simulink model "CIM_HA_Basic"  (R2016b)
settings: Solver=FixedStepDiscrete  StartTime=0.0  StopTime=10.0  FixedStep=TimeSteps.ModelStep  RelTol=1e-3
InitFcn:
  | BusInit;
undefined symbols (not defined in the file): Mechanical, Motor, TimeSteps
libraries: simulink x1
settings Model: Creator=KIRTACA  LastModifiedBy=KIRTACA

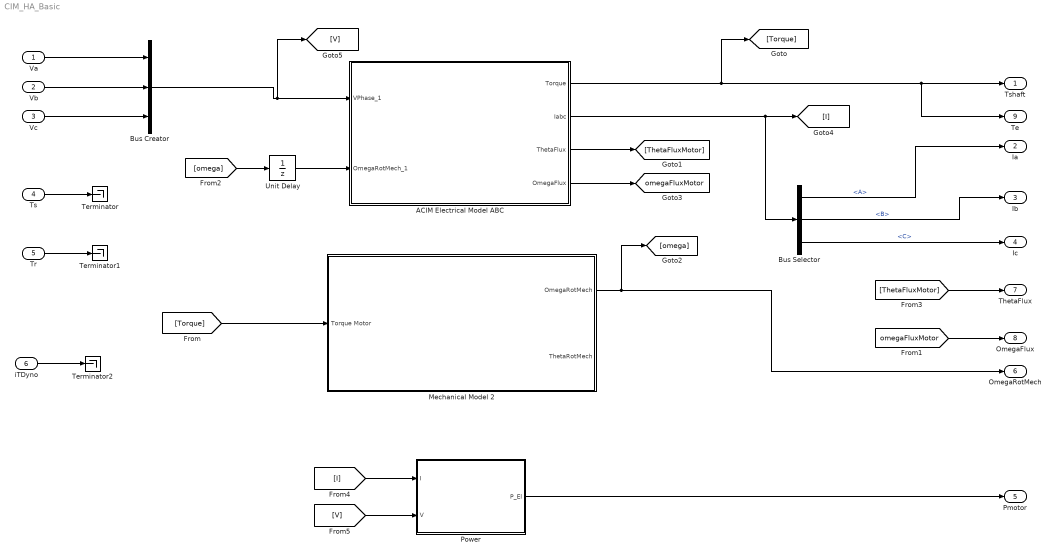
== system CIM_HA_Basic ==
  Va : Inport
  Vb : Inport  Port=2
  Vc : Inport  Port=3
  Ts : Inport  Port=4
  Tr : Inport  Port=5
  iTDyno : Inport  Port=6
  "ACIM Electrical Model ABC " : Subsystem  SystemSampleTime=Ts1  mask(ACIM_ABC){Rs=(Motor.Electrical.Rs)/(Motor.Electrical.Conn), Rr=(Motor.Electrical.Rr)/(Motor.Electrical.Conn), Ls=(Motor.Electrical.Ls)/(Motor.Electrical.Conn), Lr=(Motor.Electrical.Lr)/(Motor.Electrical.Conn), Lm=(Motor.Electrical.Lm)/(Motor.Electrical.Conn), p=Motor.Electrical.p, Ts=TimeSteps.ModelStep, Ts1=0.000125}
      mask prompts: Rs "Rs [Ohm]"; Rr "Rr [Ohm]"; Ls "Ls [H]"; Lr "Lr [H]"; Lm "Lm [H]"; Ts "Sample Time [s]"; Ts1 "Simulink:blkprm_prompts:AllBlksSampleTime"
      mask help:
      | The block implements the ACIM Electrical Model equations.
      | Input:
      | -Vphase_1: voltages applied to the motor;
      | -OmegaRotMech: mechanical rotor rotational speed;
      | Output:
      | -Torque: motor torque;
      | -Iabc: motor measured currents;
      | -OmegaFlux:
      | -ThetaFlux: angle obtained from OmegaFlux
      mask init:
      | params.Rs = Rs;
      | params.Rr = Rr;
      | params.Ls = Ls;
      | params.Lr = Lr;
      | params.Lm = Lm;
      | params.p  = p;
      | params.Ts = Ts;
      | 
      | TsACIM_ABC = Ts;
      mask Help: file:///C:\MotorControlLibrary\help/ACIM_ABC.html
      mask TypeOptions Ts1: SystemSampleTime
      mask Callback Ts1: set_param(gcb,'Ts1',num2str(eval(get_param(gcb,'Ts'))));
      mask DialogControl DescGroupVar Prompt: ACIM Electrical Model (ABC-Axis)
      mask DialogControl DescTextVar Prompt: %<MaskDescription
  Bus Creator : BusCreator  Inputs=3
  Bus Selector : BusSelector  OutputSignals=A,B,C
  Mechanical Model 2 : Subsystem  mask{TR=Motor.Mechanical.TR, M_D=Mechanical.M_D, M=Mechanical.M, R_J=Mechanical.R_J, R_Drum=Mechanical.R_Drum, InitialSpeed=0, InitialPosition=0, M_Cr=Mechanical.m_unb, R_Cr=Mechanical.r_unb, Ad=(Mechanical.damp*2*pi()*1000)/60, Ts=TimeSteps.ModelStep}
      mask prompts: TR "Transmission Ratio"; M_D "Weight Drum [Kg]"; M "Weight Inertial mass [Kg]"; R_J "Thick Inertial mass [m]"; R_Drum "Drum Radius [m]"; InitialSpeed "Initial Speed  [rad/s]"; InitialPosition "Initial Position [del_el]"; M_Cr "Weight Unbalance Load [Kg]"; R_Cr "Radius Unbalance Load [m]"; Ad "Dynamic Friction [Nm/rpm_D*1000]"; Ts "Ts [s]"
      mask init:
      | params.J = 1/2*(M_D+M)*(R_Drum^2 + (R_Drum-R_J)^2);
      | params.Ts = Ts;
      | J = 1/2*(M_D+M)*(R_Drum^2 + (R_Drum-R_J)^2);
  Power : MATLAB Function  TreatAsAtomicUnit=on
  Terminator : Terminator
  Terminator1 : Terminator
  Terminator2 : Terminator
  Unit Delay : UnitDelay  SampleTime=-1
  Tshaft : Outport
  Ia : Outport  Port=2
  Ib : Outport  Port=3
  Ic : Outport  Port=4
  Pmotor : Outport  Port=5
  OmegaRotMech : Outport  Port=6
  ThetaFlux : Outport  Port=7
  OmegaFlux : Outport  Port=8
  Te : Outport  Port=9
  tag scope: omegaFluxMotor=global
  wires:
  [Torque] -> Mechanical Model 2/1(Torque Motor)
  Mechanical Model 2/1(OmegaRotMech) -> [omega], OmegaRotMech/1
  Va/1 -> Bus Creator/1
  Vb/1 -> Bus Creator/2
  Vc/1 -> Bus Creator/3
  Ts/1 -> Terminator/1
  Tr/1 -> Terminator1/1
  Bus Selector/1 -> Ia/1  "<A>"
  Bus Selector/2 -> Ib/1  "<B>"
  Bus Selector/3 -> Ic/1  "<C>"
  [ThetaFluxMotor] -> ThetaFlux/1
  [omegaFluxMotor] -> OmegaFlux/1
  Power/1(P_El) -> Pmotor/1
  [I] -> Power/1(I)
  [V] -> Power/2(V)
  Bus Creator/1 -> [V], "ACIM Electrical Model ABC "/1(VPhase_1)
  "ACIM Electrical Model ABC "/1(Torque) -> [Torque], Te/1, Tshaft/1
  "ACIM Electrical Model ABC "/2(Iabc) -> [I], Bus Selector/1
  "ACIM Electrical Model ABC "/3(ThetaFlux) -> [ThetaFluxMotor]
  "ACIM Electrical Model ABC "/4(OmegaFlux) -> [omegaFluxMotor]
  iTDyno/1 -> Terminator2/1
  Unit Delay/1 -> "ACIM Electrical Model ABC "/2(OmegaRotMech_1)
  [omega] -> Unit Delay/1

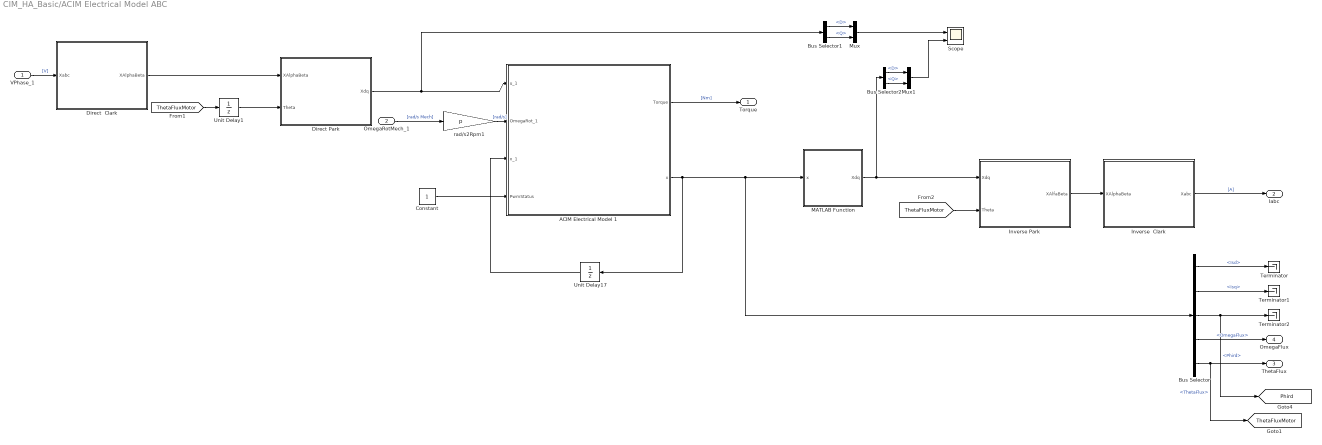
== system CIM_HA_Basic/ACIM Electrical Model ABC  ==
  VPhase_1 : Inport  OutDataTypeStr=Bus: XabcBus
  OmegaRotMech_1 : Inport  Port=2
  ACIM Electrical Model 1 : MATLAB Function  TreatAsAtomicUnit=on  SystemSampleTime=SystemSampleTime  mask{SystemSampleTime=TsACIM_ABC}
      mask prompts: SystemSampleTime "Simulink:blkprm_prompts:AllBlksSampleTime"
  Bus Selector : BusSelector  OutputSignals=Isd,Isq,Phird,OmegaFlux,ThetaFlux
  Bus Selector1 : BusSelector  OutputSignals=D,Q
  Bus Selector2 : BusSelector  OutputSignals=D,Q
  Constant : Constant
  "Direct  Clark  " : MATLAB Function  TreatAsAtomicUnit=on  SystemSampleTime=SystemSampleTime  mask{SystemSampleTime=-1}
      mask prompts: SystemSampleTime "Simulink:blkprm_prompts:AllBlksSampleTime"
  Direct Park : MATLAB Function  TreatAsAtomicUnit=on  SystemSampleTime=SystemSampleTime  mask{SystemSampleTime=-1}
      mask prompts: SystemSampleTime "Simulink:blkprm_prompts:AllBlksSampleTime"
  "Inverse  Clark  " : MATLAB Function  TreatAsAtomicUnit=on  SystemSampleTime=SystemSampleTime  mask{SystemSampleTime=-1}
      mask prompts: SystemSampleTime "Simulink:blkprm_prompts:AllBlksSampleTime"
  "Inverse Park " : MATLAB Function  TreatAsAtomicUnit=on  SystemSampleTime=SystemSampleTime  mask{SystemSampleTime=-1}
      mask prompts: SystemSampleTime "Simulink:blkprm_prompts:AllBlksSampleTime"
  MATLAB Function : MATLAB Function  TreatAsAtomicUnit=on
  Mux : Mux  Inputs=2
  Mux1 : Mux  Inputs=2
  Scope : Scope  NumInputPorts=2
  Terminator : Terminator
  Terminator1 : Terminator
  Terminator2 : Terminator
  Unit Delay1 : UnitDelay  SampleTime=-1
  Unit Delay17 : UnitDelay  SampleTime=-1
  rad/s2Rpm1 : Gain  Gain=p
  Torque : Outport
  Iabc : Outport  Port=2  OutDataTypeStr=Bus: XabcBus
  ThetaFlux : Outport  Port=3
  OmegaFlux : Outport  Port=4
  tag scope: Phird=global, ThetaFluxMotor=global
  wires:
  "Inverse Park "/1(XAlfaBeta) -> "Inverse  Clark  "/1(XAlphaBeta)
  Bus Selector/5 -> ThetaFlux/1, [ThetaFluxMotor]  "<ThetaFlux>"
  Bus Selector/4 -> OmegaFlux/1  "<OmegaFlux>"
  rad/s2Rpm1/1 -> ACIM Electrical Model 1/2(OmegaRot_1)  "[rad/s]"
  Direct Park/1(Xdq) -> Bus Selector1/1, ACIM Electrical Model 1/1(u_1)
  Bus Selector/3 -> [Phird], Terminator2/1  "<Phird>"
  Bus Selector/2 -> Terminator1/1  "<Isq>"
  Bus Selector/1 -> Terminator/1  "<Isd>"
  MATLAB Function/1(Xdq) -> Bus Selector2/1, "Inverse Park "/1(Xdq)
  [ThetaFluxMotor] -> "Inverse Park "/2(Theta)
  [ThetaFluxMotor] -> Unit Delay1/1
  Unit Delay17/1 -> ACIM Electrical Model 1/3(x_1)
  Unit Delay1/1 -> Direct Park/2(Theta)
  "Direct  Clark  "/1(XAlphaBeta) -> Direct Park/1(XAlphaBeta)
  VPhase_1/1 -> "Direct  Clark  "/1(Xabc)  "[V]"
  "Inverse  Clark  "/1(Xabc) -> Iabc/1  "[A]"
  OmegaRotMech_1/1 -> rad/s2Rpm1/1  "[rad/s Mech]"
  ACIM Electrical Model 1/1(Torque) -> Torque/1  "[Nm]"
  ACIM Electrical Model 1/2(x) -> MATLAB Function/1(x), Bus Selector/1, Unit Delay17/1
  Constant/1 -> ACIM Electrical Model 1/4(PwmStatus)
  Bus Selector1/2 -> Mux/2  "<Q>"
  Bus Selector1/1 -> Mux/1  "<D>"
  Mux/1 -> Scope/1
  Bus Selector2/2 -> Mux1/2  "<Q>"
  Bus Selector2/1 -> Mux1/1  "<D>"
  Mux1/1 -> Scope/2

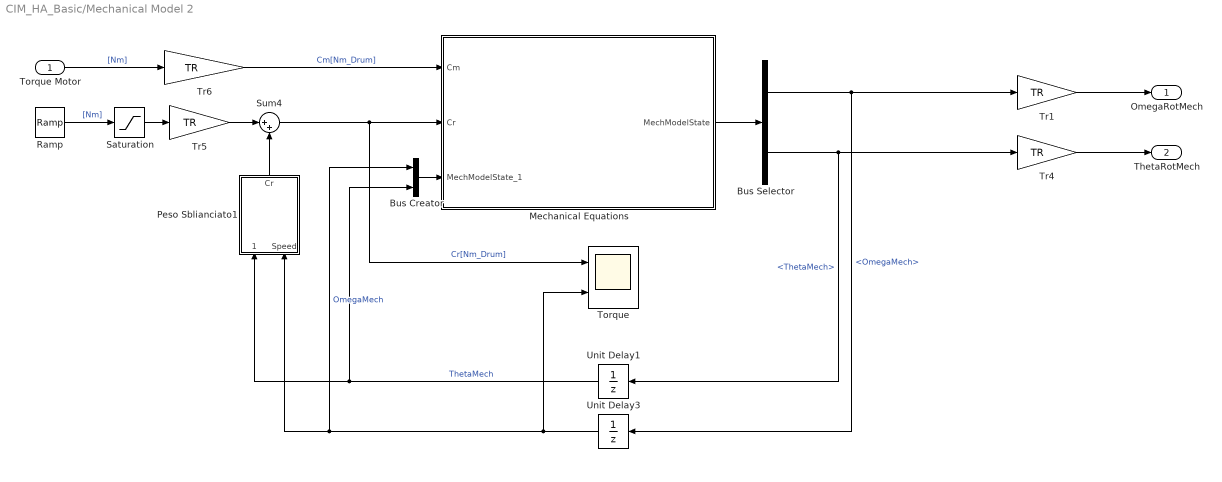
== system CIM_HA_Basic/Mechanical Model 2 ==
  Torque Motor : Inport
  " Mechanical Equations" : MATLAB Function  TreatAsAtomicUnit=on  SystemSampleTime=Ts1  mask(MechEq){J=J, Ts=Ts, Ts1=0.000125}
      mask prompts: J "J [N/rad s ^2]"; Ts "Sample Tim [s]"; Ts1 "Simulink:blkprm_prompts:AllBlksSampleTime"
      mask help:
      | The block computes the generoc mechanical equations:
      | OmegaMech = OmegaMech_1 + Ts(Cm - Cr)/J
      | ThetaMech = ThetaMech_1 + Ts OmegaMech
      | Cm : motor torque;
      | Cr : resistive torque
      mask init:
      | params.J  = J;
      |         params.Ts = Ts;
  Bus Creator : BusCreator  Inputs=2  OutDataTypeStr=Bus: Mech1stateBus
  Bus Selector : BusSelector  OutputSignals=OmegaMech,ThetaMech
  Peso Sblianciato1 : Subsystem  mask{M_Cr=M_Cr, R_Cr=R_Cr, Ad=Ad}
      mask prompts: M_Cr "Massa Peso Sblianciato [Kg]"; R_Cr "Raggio Peso Sbilanciato [m]"; Ad "Attrito Dinamico [Nm/rpm_D*100]"
  Ramp : simulink/Sources/Ramp  slope=0.4  start=0.7  X0=0
  Saturation : Saturate  UpperLimit=0  LowerLimit=0
  Sum4 : Sum  Inputs=|++
  Torque : Scope  NumInputPorts=2
  Tr{1,4..6} (4 alike) : Gain  Gain=TR
  Unit Delay1 : UnitDelay  InitialCondition=InitialPosition/Motor.Electrical.p/Motor.Mechanical.TR/180*pi  SampleTime=Ts
  Unit Delay3 : UnitDelay  InitialCondition=InitialSpeed  SampleTime=Ts
  OmegaRotMech : Outport
  ThetaRotMech : Outport  Port=2
  wires:
  Ramp/1 -> Saturation/1  "[Nm]"
  Torque Motor/1 -> Tr6/1  "[Nm]"
  Tr1/1 -> OmegaRotMech/1
  Tr4/1 -> ThetaRotMech/1
  Peso Sblianciato1/1(Cr) -> Sum4/2
  Saturation/1 -> Tr5/1
  Sum4/1 -> Torque/1, " Mechanical Equations"/2(Cr)  "Cr[Nm_Drum]"
  Tr6/1 -> " Mechanical Equations"/1(Cm)  "Cm[Nm_Drum]"
  Unit Delay1/1 -> Bus Creator/2, Peso Sblianciato1/1(Position)  "ThetaMech"
  Unit Delay3/1 -> Torque/2, Bus Creator/1, Peso Sblianciato1/2(Speed)  "OmegaMech"
  Bus Creator/1 -> " Mechanical Equations"/3(MechModelState_1)
  " Mechanical Equations"/1(MechModelState) -> Bus Selector/1
  Bus Selector/1 -> Unit Delay3/1, Tr1/1  "<OmegaMech>"
  Bus Selector/2 -> Unit Delay1/1, Tr4/1  "<ThetaMech>"
  Tr5/1 -> Sum4/1

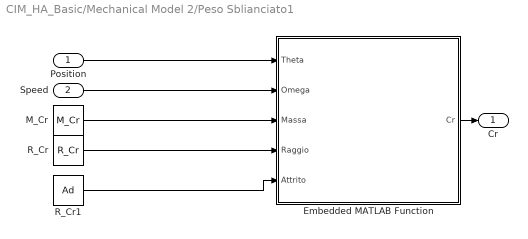
== system CIM_HA_Basic/Mechanical Model 2/Peso Sblianciato1 ==
  Position : Inport
  Speed : Inport  Port=2
  Embedded MATLAB Function : MATLAB Function  TreatAsAtomicUnit=on
  M_Cr : Constant  Value=M_Cr
  R_Cr : Constant  Value=R_Cr
  R_Cr1 : Constant  Value=Ad
  Cr : Outport
  wires:
  Embedded MATLAB Function/1(Cr) -> Cr/1
  Speed/1 -> Embedded MATLAB Function/2(Omega)
  M_Cr/1 -> Embedded MATLAB Function/3(Massa)
  R_Cr/1 -> Embedded MATLAB Function/4(Raggio)
  R_Cr1/1 -> Embedded MATLAB Function/5(Attrito)
  Position/1 -> Embedded MATLAB Function/1(Theta)

== matlab function CIM_HA_Basic/ACIM Electrical Model ABC /ACIM Electrical Model 1 ==
  data: Torque output; u_1 input Bus: XdqBus; OmegaRot_1 input; params parameter Bus: ACIMparamsBus; x_1 input Bus: ACIMstateBus; x output Bus: ACIMstateBus; PwmStatus input
function [Torque,x]  = ACIM_ElectricalModel(u_1,OmegaRot_1,params,x_1,PwmStatus)
%#codegen

Rs = params.Rs;
Rr = params.Rr;
Ls = params.Ls;
Lr = params.Lr;
Lm = params.Lm;
p  = params.p;
Ts = params.Ts;

R = Rs+ Lm^2*Rr/Lr^2;
L = (Lr*Ls-Lm^2)/Lr;

if (PwmStatus == 0)
    % Pwm is switched off
    x.Isd = 0;
    x.Isq = 0;
    x.Phird = 0;
else
    % Pwm is switched on
    x.Isd    = (1-(R*Ts)/L)*x_1.Isd+Ts*x_1.OmegaFlux*x_1.Isq+(Lm*Rr*Ts)/(L*Lr^2)*x_1.Phird+Ts/L*u_1.D;
    x.Isq    = (1-(R*Ts)/L)*x_1.Isq-Ts*x_1.OmegaFlux*x_1.Isd-((Lm*Ts)/(L*Lr))*OmegaRot_1*x_1.Phird+Ts/L*u_1.Q;
    x.Phird  = (1-(Rr*Ts)/Lr)*x_1.Phird+(Lm*Rr*Ts)/Lr*x_1.Isd;
end

num = (x_1.Isq*Lm*Rr);
den =(Lr*x_1.Phird);

Threshold = 300*2*pi;

if den == 0
    
    x.OmegaFlux = 0;
    x.ThetaFlux = 0;
    x_1.ThetaFlux = 0;
else

    OmegaFlux1 = num/den;
    
    if abs(OmegaFlux1) > Threshold
        
        if(OmegaFlux1 > 0)
 
            OmegaFlux1 = Threshold;
        else
            OmegaFlux1 = -Threshold;
        end    
    end
        x.OmegaFlux= OmegaFlux1 + OmegaRot_1;

end

x.ThetaFlux = x_1.ThetaFlux + Ts*x.OmegaFlux;

if(x.Phird<-0.05) && (x.Isd < -2.0)
    
    x.ThetaFlux = x.ThetaFlux + pi;
    x.Isd = -x.Isd; 
    x.Isq = -x.Isq;
    x.Phird = -x.Phird;
end

Torque = 1.5*p*Lm/Lr*(x.Isq*x.Phird);

== matlab function CIM_HA_Basic/ACIM Electrical Model ABC /Inverse  Clark   ==
  data: XAlphaBeta input Bus: XAlphaBetaBus; Xabc output Bus: XabcBus
function Xabc = InverseClark(XAlphaBeta)

Xabc.A = XAlphaBeta.Alpha;
Xabc.B = 0.5*(-XAlphaBeta.Alpha + sqrt(3)*XAlphaBeta.Beta);
Xabc.C = 0.5*(-XAlphaBeta.Alpha - sqrt(3)*XAlphaBeta.Beta);

== matlab function CIM_HA_Basic/ACIM Electrical Model ABC /Inverse Park  ==
  data: XAlfaBeta output Bus: XAlphaBetaBus; Xdq input Bus: XdqBus; Theta input
function XAlfaBeta = InversePark(Xdq,Theta)
%#codegen
XAlfaBeta.Alpha = Xdq.D*cos(Theta)- Xdq.Q*sin(Theta);
XAlfaBeta.Beta  = Xdq.D*sin(Theta)+ Xdq.Q*cos(Theta);

== matlab function CIM_HA_Basic/ACIM Electrical Model ABC /Direct  Clark   ==
  data: XAlphaBeta output Bus: XAlphaBetaBus; Xabc input Bus: XabcBus
function XAlphaBeta = DirectClark(Xabc)

XAlphaBeta.Alpha = Xabc.A;
XAlphaBeta.Beta =  sqrt(3)/3*(Xabc.A+2*Xabc.B);

== matlab function CIM_HA_Basic/ACIM Electrical Model ABC /Direct Park ==
  data: XAlphaBeta input Bus: XAlphaBetaBus; Xdq output Bus: XdqBus; Theta input
function Xdq = DirectPark(XAlphaBeta,Theta)

Xdq.D  =  XAlphaBeta.Alpha*cos(Theta) + XAlphaBeta.Beta*sin(Theta);
Xdq.Q  = -XAlphaBeta.Alpha*sin(Theta) + XAlphaBeta.Beta*cos(Theta);

== matlab function CIM_HA_Basic/Mechanical Model 2/ Mechanical Equations ==
  data: params parameter Bus: Mech1paramsBus; MechModelState output Bus: Mech1stateBus; Cm input; Cr input; MechModelState_1 input Bus: Mech1stateBus
function MechModelState  = MechanicalEquations(params,Cm, Cr, MechModelState_1)

Ts = params.Ts;
J  = params.J;
    
MechModelState.OmegaMech = MechModelState_1.OmegaMech + Ts/J*(Cm - Cr);
MechModelState.ThetaMech = MechModelState_1.ThetaMech + Ts*MechModelState.OmegaMech;

== matlab function CIM_HA_Basic/ACIM Electrical Model ABC /MATLAB Function ==
  data: x input Bus: ACIMstateBus; Xdq output Bus: XdqBus
function Xdq  = BusCreation(x)
Xdq.D = x.Isd;
Xdq.Q = x.Isq;

== matlab function CIM_HA_Basic/Power ==
  data: I input Bus: XabcBus; P_El output; V input Bus: XabcBus
function P_El = ElectricalPower(I,V)
%#codegen

P_El = (V.A * I.A + V.B * I.B + V.C * I.C);

== matlab function CIM_HA_Basic/Mechanical Model 2/Peso Sblianciato1/Embedded MATLAB Function ==
  data: Theta input; Omega input; Cr output; Massa input; Raggio input; Attrito input
function Cr = PesoSbilanciato(Theta, Omega, Massa, Raggio, Attrito)
%#eml
g = 9.81;

Cr = Massa*Raggio*g*sin(Theta) + Attrito*Omega*(60/(2*pi)/1000);
